simulink model "TP3combine"  (R2017b)
settings: Solver=VariableStepAuto  StartTime=0.0  StopTime=10.0  RelTol=1e-3
values from neighbouring files (symbols this model uses):
  A = [1 dt;0 1]    [TP3Combined_Main.m]    (also in TP3DC_Main.m; TP3Q3_Main.m)
  B = [dt*dt/2;dt]    [TP3Combined_Main.m]    (also in TP3DC_Main.m; TP3Q3_Main.m)
  dt = 0.001    [TP3Au422_Main.m]    (also in TP3Combined_Main.m; TP3DC_Main.m; TP3Q3_Main.m)
  F_dis1 = 150    [TP3Au422_Main.m]    (also in TP3Combined_Main.m = 0; TP3DC_Main.m; TP3Q3_Main.m = 0)
  F_dis2 = -107.5    [TP3Au422_Main.m]    (also in TP3Combined_Main.m = 0; TP3DC_Main.m; TP3Q3_Main.m = 0)
  H = [1 0;0 1]    [TP3Combined_Main.m]    (also in TP3DC_Main.m; TP3Q3_Main.m)
  Kd = 5    [TP3Au422_Main.m]    (also in TP3Combined_Main.m = 3; TP3DC_Main.m = 3; TP3Q3_Main.m = 3)
  Kp = 50    [TP3Au422_Main.m]    (also in TP3Combined_Main.m = 6; TP3DC_Main.m = 6; TP3Q3_Main.m = 6)
  m = 1    [TP3Au422_Main.m]    (also in TP3Combined_Main.m; TP3DC_Main.m; TP3Q3_Main.m)
  P0 = [VarianceU^2 0;0 VarianceA^2]    [TP3Combined_Main.m]    (also in TP3DC_Main.m; TP3Q3_Main.m)
  Q = [0.0001 0;0 2]    [TP3Combined_Main.m]    (also in TP3DC_Main.m; TP3Q3_Main.m)
  R = [VarianceU^2 0;0 0.075]    [TP3Combined_Main.m]    (also in TP3DC_Main.m; TP3Q3_Main.m)
  t_dis1 = 20    [TP3Au422_Main.m]    (also in TP3Combined_Main.m; TP3DC_Main.m; TP3Q3_Main.m)
  t_dis2 = 40    [TP3Au422_Main.m]    (also in TP3Combined_Main.m; TP3DC_Main.m; TP3Q3_Main.m)
  VarianceA = 0.075    [TP3Combined_Main.m]    (also in TP3DC_Main.m; TP3Q3_Main.m)
  VarianceU = 0.0000075    (= 7.5e-06)    [TP3Combined_Main.m]    (also in TP3DC_Main.m; TP3Q3_Main.m)
  xp0 = 0    [TP3Combined_Main.m]    (also in TP3DC_Main.m; TP3Q3_Main.m)
  xv0 = 0    [TP3Combined_Main.m]    (also in TP3DC_Main.m; TP3Q3_Main.m)
  zd = 2    [TP3Au422_Main.m]    (also in TP3Combined_Main.m; TP3DC_Main.m; TP3Q3_Main.m)
libraries: dspsrcs4 x3
settings Model: Creator=Huynh  LastModifiedBy=Huynh

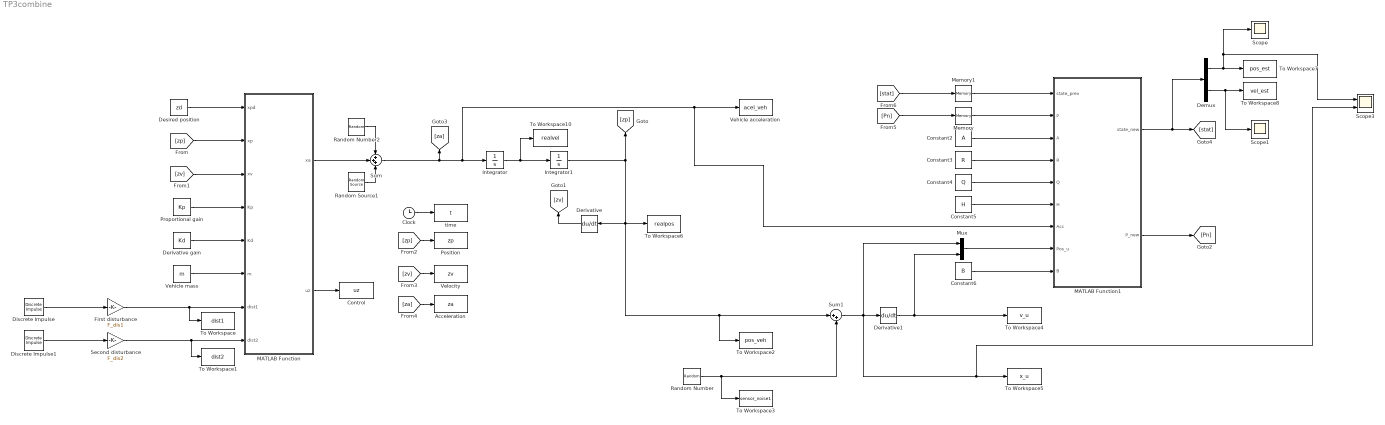
== system TP3combine ==
  Acceleration : ToWorkspace  VariableName=za  SampleTime=dt
  Clock : Clock
  Constant2 : Constant  Value=A
  Constant3 : Constant  Value=R
  Constant4 : Constant  Value=Q
  Constant5 : Constant  Value=H
  Constant6 : Constant  Value=B
  Control : ToWorkspace  VariableName=uz  SampleTime=dt
  Demux : Demux  Outputs=2
  Derivative : Derivative
  Derivative gain : Constant  Value=Kd
  Derivative1 : Derivative
  Desired position : Constant  Value=zd
  Discrete Impulse : dspsrcs4/Discrete  Impulse  Delay=t_dis1/dt  SampleTime=dt  FrameSample=1  OutputFrames=off  dataType=double  isSigned=on  wordLen=16  udDataType=sfix(16)  fracBitsMode=Best precision  numFracBits=15  OutDataTypeStr=double  LastOutDataTypeStr=double
  Discrete Impulse1 : dspsrcs4/Discrete  Impulse  Delay=t_dis2/dt  SampleTime=dt  FrameSample=1  OutputFrames=off  dataType=double  isSigned=on  wordLen=16  udDataType=sfix(16)  fracBitsMode=Best precision  numFracBits=15  OutDataTypeStr=double  LastOutDataTypeStr=double
  First disturbance : Gain  Gain=F_dis1
  Integrator : Integrator
  Integrator1 : Integrator
  MATLAB Function : MATLAB Function  TreatAsAtomicUnit=on
  MATLAB Function1 : MATLAB Function  TreatAsAtomicUnit=on
  Memory : Memory  InitialCondition=P0
  Memory1 : Memory  InitialCondition=[xp0;xv0]
  Mux : Mux  Inputs=2
  Position : ToWorkspace  VariableName=zp  SampleTime=dt
  Proportional gain : Constant  Value=Kp
  Random Number : RandomNumber  Variance=VarianceU  SampleTime=dt
  Random Number2 : RandomNumber  Variance=VarianceA  SampleTime=dt
  Random Source1 : dspsrcs4/Random Source  SrcType=Uniform  NormMethod=Ziggurat  CltLength=12  MinVal=Min  MaxVal=Max  MeanVal=0  VarVal=1  RepMode=Not repeatable  rawSeed=1  IsInherit=off  SampMode=Discrete  SampTime=Bias_Sample_time  SampFrame=1  DataType=Double  OutComplex=Real  OutputFrames=off
  Scope : Scope
  Scope1 : Scope
  Scope3 : Scope  NumInputPorts=2
  Second disturbance : Gain  Gain=F_dis2
  Sum : Sum  Inputs=+++
  Sum1 : Sum  Inputs=|++
  To Workspace : ToWorkspace  VariableName=dist1  SampleTime=dt
      settings: Save2DSignal=2-D array (concatenate along first dimension)
  To Workspace1 : ToWorkspace  VariableName=dist2  SampleTime=dt
      settings: Save2DSignal=2-D array (concatenate along first dimension)
  To Workspace10 : ToWorkspace  VariableName=realvel  SampleTime=dt
      settings: Save2DSignal=2-D array (concatenate along first dimension)
  To Workspace2 : ToWorkspace  VariableName=pos_veh  SampleTime=dt
      settings: Save2DSignal=2-D array (concatenate along first dimension)
  To Workspace3 : ToWorkspace  VariableName=sensor_noise1  SampleTime=dt
      settings: Save2DSignal=2-D array (concatenate along first dimension)
  To Workspace4 : ToWorkspace  VariableName=v_u  SampleTime=dt
      settings: Save2DSignal=2-D array (concatenate along first dimension)
  To Workspace5 : ToWorkspace  VariableName=x_u  SampleTime=dt
      settings: Save2DSignal=2-D array (concatenate along first dimension)
  To Workspace6 : ToWorkspace  VariableName=realpos  SampleTime=dt
      settings: Save2DSignal=2-D array (concatenate along first dimension)
  To Workspace7 : ToWorkspace  VariableName=pos_est  SampleTime=dt
      settings: Save2DSignal=2-D array (concatenate along first dimension)
  To Workspace8 : ToWorkspace  VariableName=vel_est  SampleTime=dt
      settings: Save2DSignal=2-D array (concatenate along first dimension)
  "Vehicle acceleration " : ToWorkspace  VariableName=acel_veh  SampleTime=dt
      settings: Save2DSignal=2-D array (concatenate along first dimension)
  Vehicle mass : Constant  Value=m
  Velocity : ToWorkspace  VariableName=zv  SampleTime=dt
  time : ToWorkspace  VariableName=t  SampleTime=dt
  wires:
  Derivative/1 -> [zv]
  [zv] -> MATLAB Function/3(xv)
  Vehicle mass/1 -> MATLAB Function/6(m)
  Clock/1 -> time/1
  Derivative gain/1 -> MATLAB Function/5(Kd)
  Discrete Impulse/1 -> First disturbance/1
  [zv] -> Velocity/1
  Discrete Impulse1/1 -> Second disturbance/1
  Integrator/1 -> To Workspace10/1, Integrator1/1
  First disturbance/1 -> To Workspace/1, MATLAB Function/7(dist1)
  Second disturbance/1 -> To Workspace1/1, MATLAB Function/8(dist2)
  [za] -> Acceleration/1
  MATLAB Function/2(uz) -> Control/1
  [zp] -> Position/1
  Proportional gain/1 -> MATLAB Function/4(Kp)
  [zp] -> MATLAB Function/2(xp)
  Random Number/1 -> To Workspace3/1, Sum1/2
  [Pn] -> Memory/1
  Constant2/1 -> MATLAB Function1/3(A)
  Constant5/1 -> MATLAB Function1/6(H)
  MATLAB Function1/2(P_new) -> [Pn]
  Memory/1 -> MATLAB Function1/2(P)
  Memory1/1 -> MATLAB Function1/1(state_prev)
  Sum1/1 -> Mux/1, Scope3/2, To Workspace5/1, Derivative1/1
  Demux/2 -> Scope1/1, To Workspace8/1
  MATLAB Function1/1(state_new) -> Demux/1, [stat]
  Mux/1 -> MATLAB Function1/8(Pos_u)
  Constant6/1 -> MATLAB Function1/9(B)
  Constant3/1 -> MATLAB Function1/4(R)
  Derivative1/1 -> Mux/2, To Workspace4/1
  [stat] -> Memory1/1
  Demux/1 -> Scope3/1, Scope/1, To Workspace7/1
  Constant4/1 -> MATLAB Function1/5(Q)
  Integrator1/1 -> Sum1/1, To Workspace2/1, To Workspace6/1, Derivative/1, [zp]
  Sum/1 -> [za], MATLAB Function1/7(Acc), "Vehicle acceleration "/1, Integrator/1
  MATLAB Function/1(xa) -> Sum/2
  Random Number2/1 -> Sum/1
  Random Source1/1 -> Sum/3
  Desired position/1 -> MATLAB Function/1(xpd)

== matlab function TP3combine/MATLAB Function1 ==
  data: state_prev input; state_new output; P input; A input; R input; Q input; H input; Acc input; Pos_u input; B input; P_new output
function [state_new, P_new] = KalmanFilterWithBias(state_prev, P, A, R, Q, H, Acc, Pos_u, B) 
%% Estimation of prediction phase
state_est = A*state_prev+B*Acc;
P_est = A*P*A'+Q;
K=P_est*H'*inv(H*P_est*H'+R);

%% Correction phase
Measu=Pos_u;
state=state_est+K*(Measu-H*state_est);
P_new=(1-K*H)*P_est;

%%
state_new = state;

== matlab function TP3combine/MATLAB Function ==
  data: xpd input; xa output; xp input; xv input; Kp input; Kd input; m input; dist1 input; dist2 input; uz output
function [xa, uz] = PD(xpd, xp, xv, Kp, Kd, m, dist1, dist2) %PD Function

exp = xpd - xp; %Position error
exv = 0 - xv; %Velocity error

uz = Kp * exp + Kd * exv + 9.81 * m; %Control law equation
if uz > 20
    uz = 20;
elseif uz < -10
    uz = -10;
end
xa = (uz + dist1 + dist2 - 9.81 * m) / m ; %Acceleration update with disturbances
